simulink model "modello_robot"  (R2022b)
settings: Solver=VariableStepAuto  StartTime=0.0  StopTime=30.0  RelTol=1e-3
undefined symbols (not defined in the file or in its folder): Kk
settings Model: Creator=alexi  LastModifiedBy=alexi

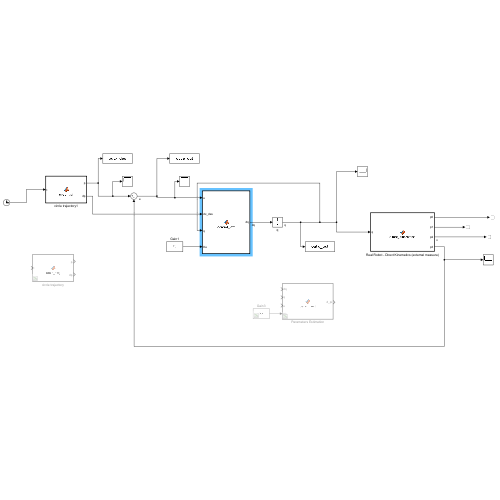
[thumbnail: Simulink's stored preview of the top-level diagram]
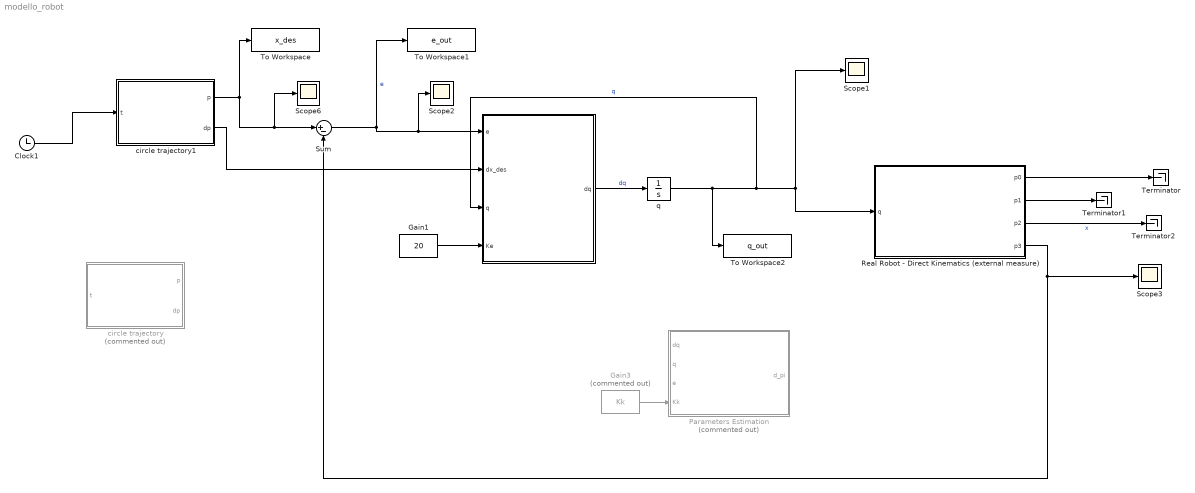
== system modello_robot ==
  " " : MATLAB Function  TreatAsAtomicUnit=on
  Clock1 : Clock
  Gain1 : Constant  Value=20
  Gain3 : Constant  Commented=on  Value=Kk
  Parameters Estimation : MATLAB Function  Commented=on  TreatAsAtomicUnit=on
  Real Robot - Direct Kinematics (external measure) : MATLAB Function  TreatAsAtomicUnit=on
  Scope{1..3,6} (4 alike) : Scope
  Sum : Sum  Inputs=|+-
  Terminator : Terminator
  Terminator1 : Terminator
  Terminator2 : Terminator
  To Workspace : ToWorkspace  VariableName=x_des  SaveFormat=Timeseries  SampleTime=-1
  To Workspace1 : ToWorkspace  VariableName=e_out  SaveFormat=Timeseries  SampleTime=-1
  To Workspace2 : ToWorkspace  VariableName=q_out  SaveFormat=Timeseries  SampleTime=-1
  circle trajectory : MATLAB Function  Commented=on  TreatAsAtomicUnit=on
  circle trajectory1 : MATLAB Function  TreatAsAtomicUnit=on
  q : Integrator  InitialCondition=[0;0;0]
  wires:
  Sum/1 -> To Workspace1/1, Scope2/1, " "/1(e)  "e"
  " "/1(dq) -> q/1  "dq"
  q/1 -> To Workspace2/1, Real Robot - Direct Kinematics (external measure)/1(q), Scope1/1, " "/3(q)  "q"
  Gain1/1 -> " "/4(Ke)
  Real Robot - Direct Kinematics (external measure)/1(p0) -> Terminator/1
  Real Robot - Direct Kinematics (external measure)/2(p1) -> Terminator1/1
  Real Robot - Direct Kinematics (external measure)/4(p3) -> Scope3/1, Sum/2
  Real Robot - Direct Kinematics (external measure)/3(p2) -> Terminator2/1  "x"
  Clock1/1 -> circle trajectory1/1(t)
  circle trajectory1/1(p) -> Scope6/1, Sum/1, To Workspace/1
  circle trajectory1/2(dp) -> " "/2(dx_des)
  Gain3/1 -> Parameters Estimation/4(Kk)

== matlab function modello_robot/  ==
  data: e input; dx_des input; q input; Ke input; dq output
function dq = control_law( e, dx_des, q , Ke )

q1 = q(1);
q2 = q(2);
q3 = q(3); 

a1 = 1;
a2 = 1;
a3 = 1;

J = [- a1*sin(q1) - a3*cos(q3)*(sin(q1+q2)) - a2*sin(q1+q2), -a3*cos(q3)*(sin(q1+q2)) - a2*sin(q1+q2), -a3*sin(q3)*(cos(q1+q2)); ...
    a1*cos(q1) + a3*cos(q3)*(cos(q1+q2)) + a2*cos(q1+q2),   a3*cos(q3)*(cos(q1+q2)) + a2*cos(q1+q2),  -a3*sin(q3)*(sin(q1+q2)); ...
    0,0,- a3*cos(q3)*(sin(q1+q2))^2 - a3*cos(q3)*(cos(q1+q2))^2];



% J = [-(a2 + a3)*(cos(q1)*sin(q2) + cos(q2)*sin(q1)) - a1*sin(q1), -(a2 + a3)*(cos(q1)*sin(q2) + cos(q2)*sin(q1)),0; ...
%         (a2 + a3)*(cos(q1)*cos(q2) - sin(q1)*sin(q2)) + a1*cos(q1),  (a2 + a3)*(cos(q1)*cos(q2) - sin(q1)*sin(q2)),0; ...
%         0,0,0];

dq = pinv(J) * (dx_des + Ke*e);
  
end

== matlab function modello_robot/Real Robot - Direct Kinematics (external measure) ==
  data: q input; p0 output; p1 output; p2 output; p3 output
function [p0, p1, p2,p3] = direct_kinematics(q)

    q1 = q(1);
    q2 = q(2);
    q3 = q(3);

    a1 = 1;
    a2 = 1;
    a3 = 1;

%     p0 = [0;0;0];
%     p1 = [a1*cos(q1); a1*sin(q1);0];
%     p2 = p1+[a2*cos(q2);a2*sin(q2);0];
%     %p2 = p1+[a2*cos(q2); a2*sin(q2);0];
%     p3 = [(a2 + a3)*(cos(q1)*cos(q2) - sin(q1)*sin(q2)) + a1*cos(q1);(a2 + a3)*(cos(q1)*sin(q2) + cos(q2)*sin(q1)) + a1*sin(q1);0];

p0 = [0;0;0];
p1 = [a1*cos(q1); a1*sin(q1);0];
p2 = p1+[a2*cos(q1+q2);a2*sin(a1+q2);0];
p3 = [a1*cos(q1) + a3*cos(q3)*(cos(q1)*cos(q2) - sin(q1)*sin(q2)) + a2*cos(q1)*cos(q2) - a2*sin(q1)*sin(q2); a1*sin(q1) + a3*cos(q3)*(cos(q1)*sin(q2) + cos(q2)*sin(q1)) + a2*cos(q1)*sin(q2) + a2*cos(q2)*sin(q1);-a3*sin(q3)];

== matlab function modello_robot/Parameters Estimation ==
  data: dq input; q input; e input; Kk input; d_pi output
function d_pi = param_est(dq, q, e, Kk)

q1 = q(1);
q2 = q(2);
q3 = q(3);

dq1 = dq(1);
dq2 = dq(2);
dq3 = dq(3);

Y = [-dq1*sin(q1), - dq1*(cos(q1)*sin(q2) + cos(q2)*sin(q1)) - dq2*(cos(q1)*sin(q2) + cos(q2)*sin(q1)), - dq1*(cos(q1)*sin(q2) + cos(q2)*sin(q1)) - dq2*(cos(q1)*sin(q2) + cos(q2)*sin(q1)); ...
      dq1*cos(q1),   dq1*(cos(q1)*cos(q2) - sin(q1)*sin(q2)) + dq2*(cos(q1)*cos(q2) - sin(q1)*sin(q2)),   dq1*(cos(q1)*cos(q2) - sin(q1)*sin(q2)) + dq2*(cos(q1)*cos(q2) - sin(q1)*sin(q2)); ...
      0,0,0];

d_pi = -Kk * Y' * e;
     
end

== matlab function modello_robot/circle trajectory1 ==
  data: t input; p output; dp output
function [p, dp] = circle_traj(t)
% Ts=1/75;
% te=(t_max/dt)/75; %Final time
% 
% x_start=[1 1 1]'; %Starting position
% v_start=[0 0 0]'; %Starting velocity
% a_start=[0 0 0]'; %Starting acceleration
% 
% %x_end=[100 45 20]'; %Final position
% %v_end=[1 5 0]'; %Final velocity
% x_end=[1.5 1.5 0.5]'; %Final position
% v_end = [0 0 0]'; %Final velocity
% a_end=[0 0 0]'; %Final acceleration
% 
% A=[te^3 te^4 te^5;
%    3*te^2 4*te^3 5*te^4;
%    6*te 12*te^2 20*te^3];
% 
% PR=zeros(6,3); %Each column is an [a0 a1 a2 a3 a4 a5]' vector
% 
% %The first three row of P comes from boundary condition (a0,a1,a2)
% PR(1,:)=[x_start(1),x_start(2),x_start(3)];
% PR(2,:)=[v_start(1),v_start(2),v_start(3)];
% PR(3,:)=[a_start(1)/2,a_start(2)/2,a_start(3)/2];
% 
% for i=1:3
% %when i = 1 we only consider x coordinate, when i = 2 we consider y
% %coordinate
% x_tend = x_end(i);
% v_tend = v_end(i);
% a_tend = a_end(i);
% M=zeros(3,1);
% M(1) = x_tend - PR(1,i) - PR(2,i)*te - PR(3,i)*(te^2);
% M(2) = v_tend - PR(2,i) - 2*PR(3,i)*te;
% M(3) = a_tend - 2*PR(3,i);
% 
% PR(4:6,i) = inv(A)*M; %the first three row of P have already been computed 
% 
% end
% i = 1;
% for t= 0:Ts:te
% x = x_start(1) + PR(2,1)*t + PR(3,1)*t^2 + PR(4,1)*t^3 + PR(5,1)*t^4 + PR(6,1)*t^5;
% y = x_start(2) + PR(2,2)*t + PR(3,2)*t^2 + PR(4,2)*t^3 + PR(5,2)*t^4 + PR(6,2)*t^5;
% z = x_start(3) + PR(2,3)*t + PR(3,3)*t^2 + PR(4,3)*t^3 + PR(5,3)*t^4 + PR(6,3)*t^5;
% 
% vx = PR(2,1) + 2*PR(3,1)*t+3*PR(4,1)*t^2 + 4*PR(5,1)*t^3 + 5*PR(6,1)*t^4;
% vy = PR(2,2) + 2*PR(3,2)*t+3*PR(4,2)*t^2 + 4*PR(5,2)*t^3 + 5*PR(6,2)*t^4;
% vz = PR(2,3) + 2*PR(3,3)*t+3*PR(4,3)*t^2 + 4*PR(5,3)*t^3 + 5*PR(6,3)*t^4;
% 
% 
% position =[x y z]';
% velocity = [vx vy vz]';
% a = [ax ay az]';
% 
% i = i+1;
% end
% p = position;
% dp = velocity; 

a = 0.2;    % Ampiezza lungo l'asse X
b = 0.1;    % Ampiezza lungo l'asse Y
p0 = [0.8;0.8;0.8];

x = a * cos(t);
y = b * sin(t);
z =  0.1 * sin(t);

p = [x y z]'+p0;

dx = -a*sin(t);
dy = b*cos(t);
dz = 0.5*cos(t);

dp = [dx dy dz]';

== matlab function modello_robot/circle trajectory ==
  data: t input; p output; dp output
function [p, dp] = circle_traj(t)

% p0 = [0.75; 0.75];
% 
% A = 0.25; % 0.25
% w = 0.5;
% 
% p =  [A*cos(w*t); A*sin(w*t)] + p0;
% dp = [-A*w*sin(w*t); A*w*cos(w*t)];


radius = 1; % Raggio della sfera
omega = 0.2; % Velocità angolare
p0 = [0.75; 0.75;1];

% Calcolo delle coordinate x, y e z sulla sfera
x = radius * cos(omega * t);
y = radius * sin(omega * t);
z = radius * sqrt(1 - x.^2 - y.^2); % Z calcolato per mantenere sulla sfera
p = [x;y;z]+p0;

dx_dt = -radius*omega*sin(omega*t);
dy_dt = radius*omega*cos(omega*t);
dz_dt = -radius*omega^2 *x *cos(omega*t) / sqrt(1 - x^2 - y^2);
dp = [dx_dt;dy_dt;dz_dt];
